simulink model "case1"  (R2024a)
settings: Solver=VariableStepAuto  StartTime=0.0  StopTime=10.0  RelTol=1e-3
settings Model: Creator=tusha  LastModifiedBy=tusha

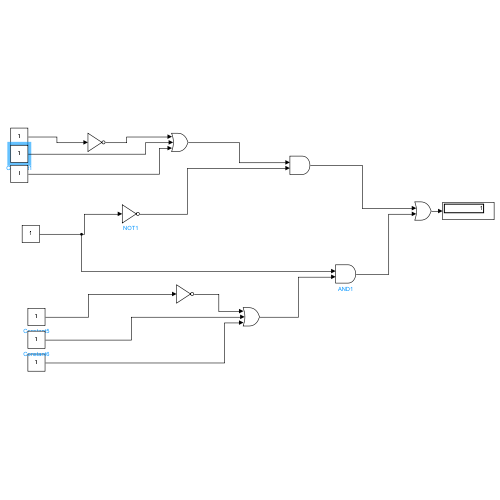
[thumbnail: Simulink's stored preview of the top-level diagram]
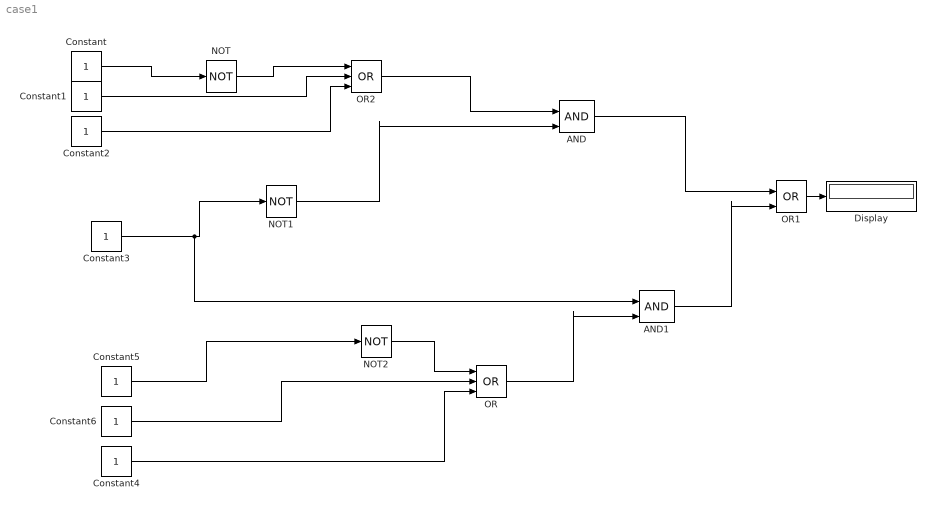
== system case1 ==
  AND : Logic  IconShape=distinctive  AllPortsSameDT=off  OutDataTypeStr=boolean
  AND1 : Logic  IconShape=distinctive  AllPortsSameDT=off  OutDataTypeStr=boolean
  Constant{,1..6} (7 alike) : Constant
  Display : Display
  NOT : Logic  Operator=NOT  IconShape=distinctive  AllPortsSameDT=off  OutDataTypeStr=boolean
  NOT1 : Logic  Operator=NOT  IconShape=distinctive  AllPortsSameDT=off  OutDataTypeStr=boolean
  NOT2 : Logic  Operator=NOT  IconShape=distinctive  AllPortsSameDT=off  OutDataTypeStr=boolean
  OR : Logic  Operator=OR  Inputs=3  IconShape=distinctive  AllPortsSameDT=off  OutDataTypeStr=boolean
  OR1 : Logic  Operator=OR  IconShape=distinctive  AllPortsSameDT=off  OutDataTypeStr=boolean
  OR2 : Logic  Operator=OR  Inputs=3  IconShape=distinctive  AllPortsSameDT=off  OutDataTypeStr=boolean
  wires:
  Constant/1 -> NOT/1
  NOT/1 -> OR2/1
  Constant1/1 -> OR2/2
  Constant2/1 -> OR2/3
  Constant3/1 -> AND1/1, NOT1/1
  NOT1/1 -> AND/2
  OR2/1 -> AND/1
  AND/1 -> OR1/1
  Constant5/1 -> NOT2/1
  NOT2/1 -> OR/1
  Constant6/1 -> OR/2
  Constant4/1 -> OR/3
  AND1/1 -> OR1/2
  OR/1 -> AND1/2
  OR1/1 -> Display/1
